simulink model "example_SQProblem"  (Simulink 7.2)
settings: Solver=VariableStepDiscrete  StartTime=0.0  StopTime=0.5  RelTol=1e-3
settings Model: Creator=jferreau  LastModifiedBy=jferreau  ExtModeAutoUpdateStatusClock=off
settings OptimizationCC: InitFltsAndDblsToZero=on
settings DebuggingCC: SaveWithParameterizedLinksMsg=none  SignalResolutionControl=TryResolveAllWithWarning
settings GRTTargetCC: TargetFcnLib=ansi_tfl_tmw.mat

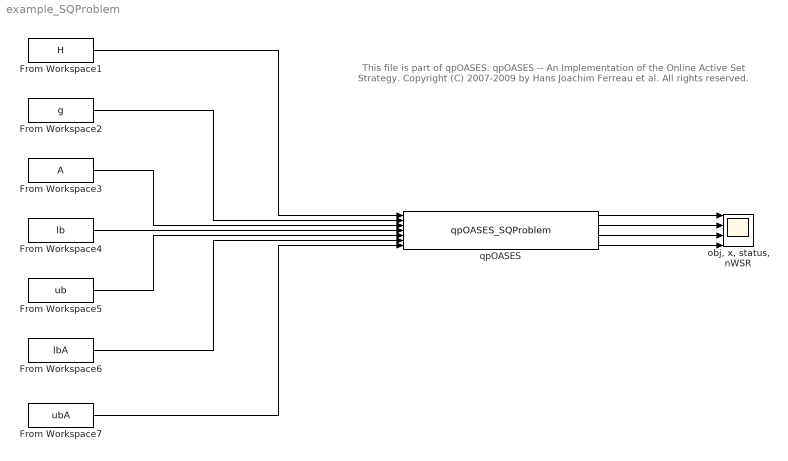
== system example_SQProblem ==
  note: This file is part of qpOASES.
      |
      | qpOASES -- An Implementation of the Online Active Set Strategy.
      | Copyright (C) 2007-2009 by Hans Joachim Ferreau et al. All rights reserved.
  From Workspace1 : FromWorkspace  VariableName=H  SampleTime=0.1  OutputAfterFinalValue=Holding final value
  From Workspace2 : FromWorkspace  VariableName=g  SampleTime=0.1  OutputAfterFinalValue=Holding final value
  From Workspace3 : FromWorkspace  VariableName=A  SampleTime=0.1  OutputAfterFinalValue=Holding final value
  From Workspace4 : FromWorkspace  VariableName=lb  SampleTime=0.1  OutputAfterFinalValue=Holding final value
  From Workspace5 : FromWorkspace  VariableName=ub  SampleTime=0.1  OutputAfterFinalValue=Holding final value
  From Workspace6 : FromWorkspace  VariableName=lbA  SampleTime=0.1  OutputAfterFinalValue=Holding final value
  From Workspace7 : FromWorkspace  VariableName=ubA  SampleTime=0.1  OutputAfterFinalValue=Holding final value
  "obj, x, status, nWSR" : Scope  NumInputPorts=4
      settings: YMin=-5~-5~-5~-5  YMax=5~5~5~5
  qpOASES : S-Function  FunctionName=qpOASES_SQProblem  EnableBusSupport=off
  wires:
  From Workspace1/1 -> qpOASES/1
  From Workspace2/1 -> qpOASES/2
  From Workspace7/1 -> qpOASES/7
  From Workspace5/1 -> qpOASES/5
  From Workspace4/1 -> qpOASES/4
  From Workspace3/1 -> qpOASES/3
  From Workspace6/1 -> qpOASES/6
  qpOASES/1 -> "obj, x, status, nWSR"/1
  qpOASES/2 -> "obj, x, status, nWSR"/2
  qpOASES/3 -> "obj, x, status, nWSR"/3
  qpOASES/4 -> "obj, x, status, nWSR"/4
